simulink model "lasim1"  (Simulink 2.09)
settings: Solver=ode45  StartTime=0.0  StopTime=7.0  RelTol=1e-3  AbsTol=1e-6
settings Model: ConsistencyChecking=off  RTWTemplateMakefile=grt_vc.tmf

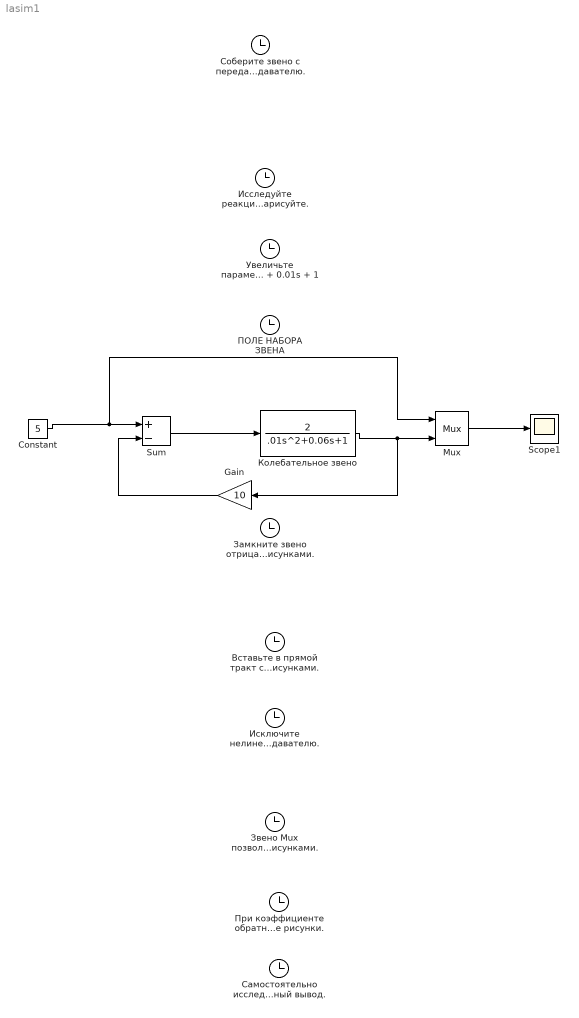
== system lasim1 ==
  Constant : Constant  Value=5
  Gain : Gain  Orientation=left  Gain=10
  Mux : Mux  Inputs=2
  Scope1 : Scope
      settings: TickLabels=on  TimeRange=auto  YMin=-5  YMax=5  SaveToWorkspace=off  SaveName=ScopeData
  Sum : Sum  Inputs=+-
  "Вставьте в прямой тракт системы перед колебательным звеном звено Dead Zone  из блока  Nonlinear.  Предлагается исследовать величину зо- ны нечувствительности на  динамические свойства  звена при  постоянном входном воздействии.  Изменять данную величину  можно при вызо- ве окна звена. Коэффициент обратной связи системы установите равным 5. Величину зоны нечувствительности последовательно задайте рав- ной  0.1;  0.7; 1.5. Сделайте вывод о влиянии этого параметра, обосновав его соответствующими рисунками." : Clock
  "Замкните звено отрицательной (!) обратной связью, используя звено  Sum  блока Linear. Для задания коэффициента обратной связи надо ис- пользовать звено   Gain  из блока  Linear.  Это звено отличает направленность, и в данном случае его следует развернуть на 180 градусов. Для этого щелкните \"мышью\" на слове Format в меню файла  lasim1 и в выпавшем меню выберите опцию (т.е. щелкните джойстиком) Rotate Blok. При этом звено повернется на 90 градусов. После этого повторите данные действия еще раз. Примечание: перед поворотом звено долж- но остаться (после переноса) отмеченным  черными точками по углам поля. Коэффициент обратной связи установите равным 1.5, 5 и 10, по- следовательно вызывая окно параметров звена. Как изменяется реакция звена с обратной связью на то же самое входное воздействие? Вы-  вод в отчете подтвердите соответствующими рисунками." : Clock
  "Звено Mux позволит выводить сразу два сигнала, что позволяет оценить наличие сдвига фаз сигналов. Самостоятельно исследуйте следую- щий вопрос: как влияет на амплитуду и фазу выходного сигнала коэффициент обратной связи системы с параметром затухания 0.05? Коэф- фициент обратной связи изменяйте по значениям  2; 1.5; 1.0; 0.8; 0.6; 0.5. (Для необходимых изменений параметров \"экрана\" виртуального ос- циллографа обратитесь к преподавателю). Ответ подтвердите соответствующими рисунками." : Clock
  "Исключите нелинейный элемент из системы. Для этого щелкните \"мышью\" в поле обозначения элемента, затем  (джойстиком)  вызовите опцию Edit  и в открывшемся окне щелкните \"мышью\" в строке Cut ; затем аналогично исключите ненужные стрелки и соедините блоки Sum и Transfer Fcn новой стрелкой. Вставьте между выходом звена и осциллографом Scope звено Mux из блока Connections библиотеки. Вызвав окно этого зве- на, установите число его входов равным 2. Соедините выход звена Transfer Fcn с одним из входов звена Mux. Замените звено постоянного воз- действия Constant на звено гармонического воздействия Sine Wave. Амплитуду воздействия установите равной 2.7, частоту - 10. Выход звена Sine Wave соедините с положительным входом звена Sum, а также со вторым входом звена Mux. В случае затруднений сообщите преподавателю." : Clock
  "Исследуйте реакцию звена на постоянное входное воздействие. Для этого подключите к его входу из блока Sources звено Constant, а также осциллограф Scope из блока Sinks. Величину входного воздействия можно задать в окне звена Constant в строке Constant Value . Значение воздействия выберите произвольно в диапазоне  2.0 - 5.0 Реакцию звена зарисуйте." : Clock
  Колебательное звено : TransferFcn  Numerator=[2]  Denominator="[.01 0.06  1 ]"
  "ПОЛЕ НАБОРА ЗВЕНА                                                                                                                                                    " : Clock
  "При коэффициенте обратной связи, равным 2, исследуйте влияние частоты входного воздействия в диапазоне чисел 16 - 28 с шагом 2 (в стро- ке  Frequency). Определите экспериментально частоту воздействия, при которой реакцию системы отличает наибольшая амплитуда. Эту час- тоту назовем резонансной . Чему равен тогда максимальный коэффициент усиления системы? Сделайте необходимые рисунки." : Clock
  Самостоятельно исследуйте вопрос: как повлияет увеличение коэффициента обратной связи на величину резонансной частоты. Для этого про- ведите эксперимент  при значениях коэффициента 0.8 и 5. Сделайте обобснованный вывод. : Clock
  "Соберите звено с передаточной функцией колебательного звена.  Для этого перенесите в поле  набора  звена из блока  Linear  звено Transfer Fcn, после чего дважды щелкните \"мышью\" на поле перенесенного звена. При этом откроется окно задания параметров звена. Строка  \"Numerator\" служит для задания коэффициентов некоторого полинома P(s) числителя. Например, для задания в числителе по- линома  2(s^2) +.5s +3 необходимо в строке \"Numerator\" задать последовательность чисел   2  .5  3.  Для задания отдельного коэффи- циента, таким образом, нужно задать только одно число.  В строке  \"Denominator\" аналогично задается полином знаменателя.  Пред- лагается выбрать следующую передаточную функцию:  W(s) = 2 / 0.01s^2 + 0.06s + 1.  Ответьте  на  вопрос: чему равен параметр зату- хания такого колебательного звена? Примечание: собранное звено может не уместиться в исходном прямоугольнике границы. В этом случае прямоугольник следует растянуть. Сообщите об этом преподавателю." : Clock
  Увеличьте параметр затухания в: 1) 0.5;  2) 2 раза. Зарисуйте реакции звена и сделайте вывод о влиянии параметра затухания на ди- намическиекие свойства колебательного звена. Теперь увеличьте постоянную времени звена в 2 раза и проведите аналогичную работу. После этого восстановите передаточную функцию звена  W(s) = 2 / 0.01s^2 + 0.01s + 1 : Clock
  wires:
  Mux/1 -> Scope1/1
  Колебательное звено/1 -> Mux/2, Gain/1
  Gain/1 -> Sum/2
  Constant/1 -> Sum/1, Mux/1
  Sum/1 -> Колебательное звено/1
